simulink model "BMSBalancingLogic"  (R2023a)
settings: Solver=FixedStepDiscrete  StartTime=0.0  StopTime=10000  RelTol=1e-3
model workspace (MAT data in the model file):
  BalNotActWait = 30
  BalOffWait = 20
  BalOnWait = 60
  TargetDeltaV = 0.00999999977648
  flgEnBalancing = 1
undefined symbols (not defined in the file): PlntBattModNumCellSer, PlntBattNumMod
settings Model: DataDictionary=VirtualVehicleTemplate.sldd  ModifiedByFormat=The MathWorks, Inc.  ExtModeTrigDuration=5  Creator=The MathWorks, Inc.  LastModifiedBy=The MathWorks, Inc.
settings SolverCC: AlgebraicLoopSolver=TrustRegion  PositivePriorityOrder=on  AutoInsertRateTranBlk=on  MaxZcPerStep=1
settings DataIOCC: ExternalInput=Battery  SaveOutput=off  SaveTime=off  SignalLoggingName=logsOut
settings OptimizationCC: BlockReduction=off  DefaultParameterBehavior=Inlined  UseFloatMulNetSlope=on  DefaultUnderspecifiedDataType=single  OptimizeBlockIOStorage=off  EnhancedBackFolding=on  PassReuseOutputArgsThreshold=0  ZeroExternalMemoryAtStartup=off  ZeroInternalMemoryAtStartup=off  EfficientFloat2IntCast=on  MaxStackSize=64  OptimizeBlockOrder=speed  DifferentSizesBufferReuse=on
settings DebuggingCC: SignalInfNanChecking=error  SaveWithParameterizedLinksMsg=none  CheckExecutionContextPreStartOutputMsg=on  IntegerOverflowMsg=error  ParameterPrecisionLossMsg=none  ParameterTunabilityLossMsg=error  UnconnectedInputMsg=warning  UnconnectedOutputMsg=warning  UnconnectedLineMsg=warning  AssertControl=DisableAll  PregeneratedLibrarySubsystemCodeDiagnostic=none  SFUnexpectedBacktrackingDiag=warning  SFNoUnconditionalDefaultTransitionDiag=warning  SFExecutionAtInitializationDiag=none  ArithmeticOperatorsInVariantConditions=warning
settings HardwareCC: ProdBitPerLong=64  ProdLongLongMode=on  ProdHWDeviceType=Intel->x86-64 (Linux 64)
settings ModelReferenceCC: EnableRefExpFcnMdlSchedulingChecks=on  ModelReferenceNumInstancesAllowed=Single  PropagateSignalLabelsOutOfModel=off
settings SFSimCC: SimUseLocalCustomCode=off  MATLABDynamicMemAlloc=off  CustomCodeUndefinedFunction=UseInterfaceOnly
settings RTWCC: GenerateReport=on  RTWUseLocalCustomCode=off  Toolchain=Simulink Real-Time Toolchain  BuildConfiguration=Faster Runs  TargetLang=C++  DLArmComputeVersion=19.05
settings CodeAppCC: ForceParamTrailComments=on  MaxIdLength=51  OperatorAnnotations=on  MangleLength=4
settings GRTTargetCC: TargetLangStandard=C++03 (ISO)  CodeInterfacePackaging=C++ class
settings ConfigComp: CovMetricSettings=dcw  CovSaveCumulativeToWorkspaceVar=on  CovSaveSingleToWorkspaceVar=on  CovExternalEMLEnable=off  CovSFcnEnable=off  DVMode=DesignErrorDetection  DVMaxProcessTime=7000  DVTestSuiteOptimization=Auto  DVDetectDeadLogic=on  DVDetectIntegerOverflow=off  DVRebuildModelRepresentation=Always

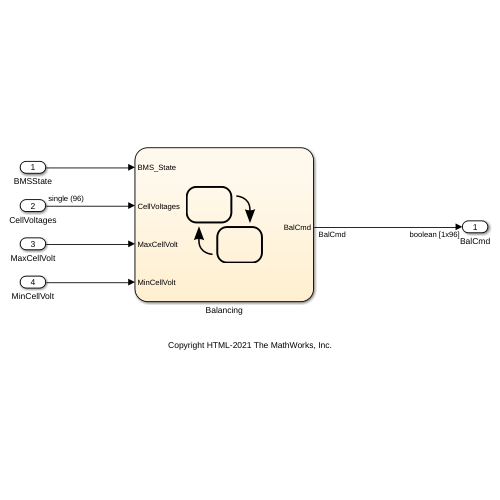
[thumbnail: Simulink's stored preview of the top-level diagram]
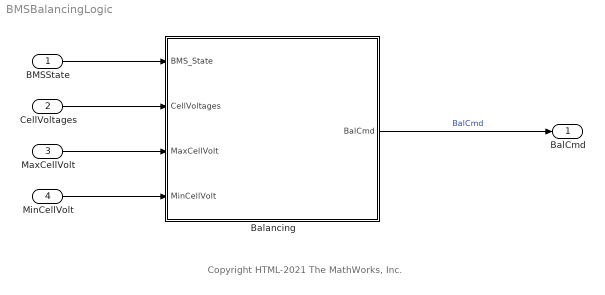
== system BMSBalancingLogic ==
  note: Copyright HTML-2021 The MathWorks, Inc.
  BMSState : Inport  PortDimensions=1  SampleTime=[5,0]
  CellVoltages : Inport  Port=2  OutDataTypeStr=single  PortDimensions=PlntBattModNumCellSer*PlntBattNumMod  SampleTime=[5,0]
  MaxCellVolt : Inport  Port=3
  MinCellVolt : Inport  Port=4
  Balancing : Stateflow chart  TreatAsAtomicUnit=on  VariantControl=(default)
  BalCmd : Outport  OutDataTypeStr=boolean  PortDimensions=[1,PlntBattModNumCellSer*PlntBattNumMod]  SampleTime=[5,0]  VectorParamsAs1DForOutWhenUnconnected=off
  wires:
  MinCellVolt/1 -> Balancing/4(MinCellVolt)
  MaxCellVolt/1 -> Balancing/3(MaxCellVolt)
  CellVoltages/1 -> Balancing/2(CellVoltages)
  Balancing/1(BalCmd) -> BalCmd/1  "BalCmd"
  BMSState/1 -> Balancing/1(BMS_State)

== stateflow chart BMSBalancingLogic/Balancing ==
  state BalancingOFF
    en:
    BalCmd(:,:) = false;
    en,du:
    DeltaCellVolt = MaxCellVolt - MinCellVolt;
  state BalancingON
    en, du:
    DeltaCellVolt = MaxCellVolt - MinCellVolt;
    state BalActive
      en, du:
      BalCmd = ((CellVoltages - MinCellVolt) > TargetDeltaV/2)';
      flgBalCompl = all(~BalCmd);
    state BalNotActive
    (default) -> BalActive
    BalNotActive -> BalActive [order 1] : [after(BalNotActWait,sec) && ...
        | DeltaCellVolt > TargetDeltaV]
    BalActive -> BalNotActive : [flgBalCompl]
  (default) -> BalancingOFF : {flgBalCompl = true;}
  BalancingOFF -> BalancingON : [flgEnBalancing && ...
      | BMS_State ~= 2 && ...
      | after(BalOffWait,sec) && ...
      | DeltaCellVolt > TargetDeltaV]
  BalancingON -> BalancingOFF : [BMS_State == 2]
      | %In Driving State
  BalNotActive -> BalancingOFF [order 2] : [after(BalOnWait,sec)]
  data: BMS_State input; CellVoltages input single; TargetDeltaV parameter; BalCmd output boolean size=[1,PlntBattModNumCellSer*PlntBattNumMod] =boolean(zeros(1,PlntBattModNumCellSer*PlntBattNumMod)); flgBalCompl local; MaxCellVolt input single; MinCellVolt input single; BalNotActWait parameter; BalOffWait parameter; BalOnWait parameter; flgEnBalancing parameter; DeltaCellVolt local single =single(0)
